simulink model "Ex_6"  (Simulink 8.0)
settings: Solver=ode45  StartTime=0.0  StopTime=10  RelTol=1e-3
settings Model: Creator=Faradars  LastModifiedBy=Faradars

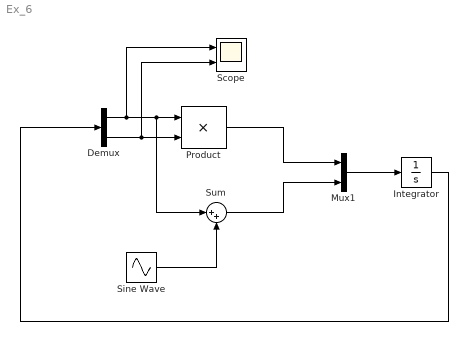
== system Ex_6 ==
  Demux : Demux  Outputs=2
  Integrator : Integrator  InitialCondition=[1e-7 0.001]
  Mux1 : Mux  Inputs=2
  Product : Product  RndMeth=Zero
  Scope : Scope  NumInputPorts=2
      settings: YMin=-5~-5  YMax=5~5
  Sine Wave : Sin  SampleTime=0
  Sum : Sum  Inputs=|++
  wires:
  Sine Wave/1 -> Sum/2
  Demux/1 -> Scope/1, Sum/1, Product/1
  Demux/2 -> Scope/2, Product/2
  Product/1 -> Mux1/1
  Sum/1 -> Mux1/2
  Mux1/1 -> Integrator/1
  Integrator/1 -> Demux/1
